simulink model "pixhawk_position_v100"  (R2016b)
settings: Solver=FixedStepAuto  StartTime=0.0  StopTime=inf  FixedStep=0.01  RelTol=1e-3
PreLoadFcn:
  | load('bus_mavlink_att_pos_mocap_t.mat');
  | load('bus_mavlink_attitude_t.mat');
  | load('bus_mavlink_heartbeat_t.mat');
  | load('bus_mavlink_raw_imu_t.mat');
  | load('bus_mavlink_set_attitude_target_t.mat');
  | load('bus_mavlink_set_mode_t.mat');
  | load('bus_mavlink_set_position_target_local_ned_t.mat');
  | 
  | load('bus_mavlink_data_stream_t.mat');
  | load('bus_mavlink_request_data_stream_t.mat');
  | load('bus_mavlink_attitude_target_t.mat');
  | load('bus_mavlink_position_target_local_ned_t.mat');
  | load('bus_mavlink_rc_channels_raw_t.mat');
  | load('bus_mavlink_rc_channels_t.mat')
libraries: dspnetwork x5, etargetslib x4, aerolibanimutils x1
settings Model: Creator=Admin  LastModifiedBy=luminghua

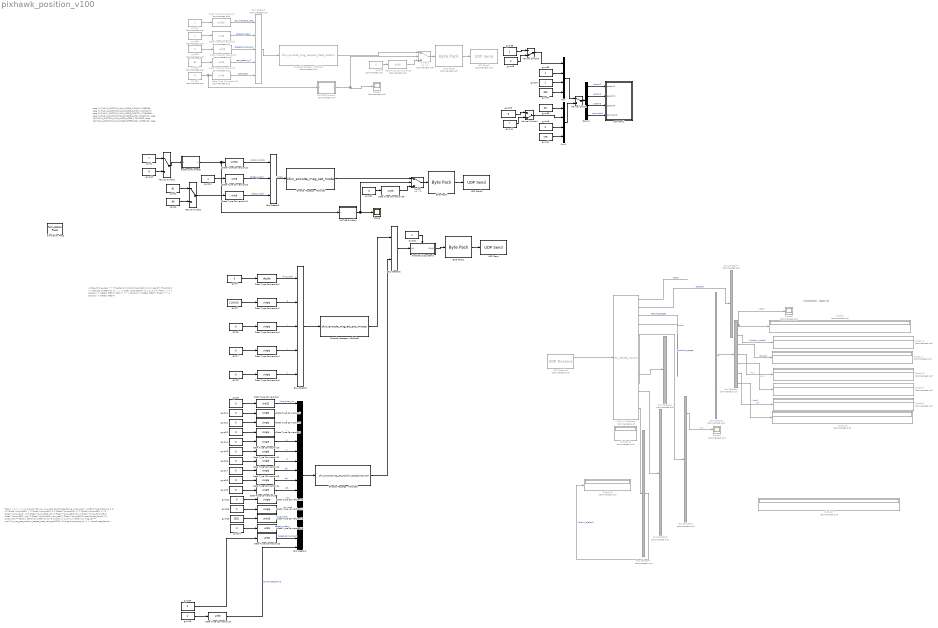
== system pixhawk_position_v100 ==
  note: case {1}%PX4_CUSTOM_MAIN_MODE_MANUAL
      |         y=65536;
      |      case {2}%PX4_CUSTOM_MAIN_MODE_ALTCTL
      |         y=131072;
      |      case {3}%PX4_CUSTOM_MAIN_MODE_POSCTL
      |         y=196608;
      |      case {4}%PX4_CUSTOM_MAIN_MODE_AUTO
      |         y=262144;
      |      case {5}%PX4_CUSTOM_MAIN_MODE_ACRO
      |         y=327680;
      |      case {6}%PX4_CUSTOM_MAIN_MODE_OFFBOARD
      |         y=393216;
      |      case {7}%PX4_CUSTOM_MAIN_MODE_STABILIZED
      |         y=458752;
      |       case {8}%PX4_CUSTOM_MAIN_MODE_RATTITUDE
  note: 不能接受数据时，查看防火墙
  note: uint64_t time_usec; /*< Timestamp (micros since boot or Unix epoch)*/
      |  float q[4]; /*< Attitude quaternion (w, x, y, z order, zero-rotation is 1, 0, 0, 0)*/
      |  float x; /*< X position in meters (NED)*/
      |  float y; /*< Y position in meters (NED)*/
      |  float z; /*< Z position in meters (NED)*/
  note: float x,y,z, vx ,vy,vz ,afx,afy,afz,yaw,yaw_rate,coordinate_frame, type_mask;
      | uint32_t time_boot_ms = 0;
      | x= (float) (*pInput[0]);
      | y = (float) (*pInput[1]);
      | z = (float) (*pInput[2]);
      | vx = (float) (*pInput[3]);
      | vy = (float) (*pInput[4]);
      | vz = (float) (*pInput[5]);
      | afx = (float) (*pInput[6]);
      | afy = (float) (*pInput[7]);
      | afz = (float) (*pInput[8]);
      | yaw = (float) (*pInput[9]);
      | yaw_rate = (float) (*pInput[10]);
      | coordinate_frame = 1;
      | type_mask = 2552;// 0001(yaw_rate) 0(yaw) 0 111(axyz) 111(vxyz) 000(xyz)
      | msg_len = mavlink_msg_set_position_target_local_ned_pack(255, 0,&msg,time_boot_ms, 1, 1, coordinate_frame, type_mask, x, y, z, vx, vy, vz, afx, afy, afz, yaw, yaw_rate);
      | ptrBuf = (uint8_T*) ssGetDWork(S,index);
      | ptrLen[index] = (real_T) mavlink_msg_to_send_buffer(ptrBuf, &msg);
      | type_mask = 1528;// 000 0(yaw_rate) 1(yaw) 0 111(axyz) 111(vxyz) 000(xyz)
      | setpoint: type_mask = 1528;// 0(idle) 0(loiter) 0(land) 0(takeoff) 0(yaw_rate) 1(yaw) 0 111(axyz) 111(vxyz) 000(xyz)
      | idle: type_mask = 34296;// 1(idle) 0(loiter) 0(land) 0(takeoff) 0(yaw_rate) 1(yaw) 0 111(axyz) 111(vxyz) 000(xyz)
      | takeoff: type_mask = 5624;// 0(idle) 0(loiter) 0(land) 1(takeoff) 0(yaw_rate) 1(yaw) 0 111(axyz) 111(vxyz) 000(xyz)
      | land: type_mask = 4856;// 0(idle) 0(loiter) 1(land) 0(takeoff) 0(yaw_rate) 1(yaw) 0 111(axyz) 111(vxyz) 000(xyz)
      |
      | yes_yaw no_yawrate
      | setpoint: type_mask = 2552;// 0(idle) 0(loiter) 0(land) 0(takeoff) 1(yaw_rate) 0(yaw) 0 111(axyz) 111(vxyz) 000(xyz)
  Bus Creator1 : BusCreator  Inputs=5  OutDataTypeStr=Bus: mavlink_att_pos_mocap_t
  Bus Creator2 : BusCreator  Inputs=2
  Bus Creator3 : BusCreator  Inputs=3  OutDataTypeStr=Bus: mavlink_set_mode_t
  Bus Creator4 : BusCreator  Inputs=16  OutDataTypeStr=Bus: mavlink_set_position_target_local_ned_t
  Bus Creator5 : BusCreator  Commented=on  Inputs=5  OutDataTypeStr=Bus: mavlink_request_data_stream_t
  Bus Creator6 : BusCreator  Commented=on  Inputs=4
  Bus Selector : BusSelector  Commented=on  OutputSignals=attitude.roll,heart.custom_mode,attitude_target.thrust,position_target.x,position_target.y,position_target.z,position_target.yaw
  Bus Selector1 : BusSelector  Commented=on  OutputSignals=time_boot_ms,q,body_roll_rate,body_pitch_rate,body_yaw_rate,thrust,type_mask
  Bus Selector2 : BusSelector  Commented=on  OutputSignals=time_boot_ms,x,y,z,vx,vy,vz,afx,afy,afz,yaw,yaw_rate,type_mask,coordinate_frame
  Bus Selector3 : BusSelector  Commented=on  OutputSignals=chan1_raw,chan2_raw,chan3_raw,chan4_raw,chan5_raw,chan6_raw,chan7_raw,chan8_raw
  Bus Selector4 : BusSelector  Commented=on  OutputSignals=chan1_scaled
  Bus Selector5 : BusSelector  Commented=on  OutputSignals=time_boot_ms,roll,pitch,yaw,rollspeed,pitchspeed,yawspeed
  Byte Pack1 : etargetslib/Byte Pack  datatypes={'uint8'}  byteAlign=1
  Byte Pack2 : etargetslib/Byte Pack  datatypes={'uint8'}  byteAlign=1
  Byte Pack3 : etargetslib/Byte Pack  Commented=on  datatypes={'uint8'}  byteAlign=1
  Data Type Conversion1 : DataTypeConversion  OutDataTypeStr=double
  Data Type Conversion{2..5,7..17} (15 alike) : DataTypeConversion  OutDataTypeStr=single
  Data Type Conversion18 : DataTypeConversion  OutDataTypeStr=uint16
  Data Type Conversion{19..21,23..24,28} (6 alike) : DataTypeConversion  OutDataTypeStr=uint8
  Data Type Conversion22 : DataTypeConversion  OutDataTypeStr=uint32
  Data Type Conversion{25..26,29..31} (5 alike) : DataTypeConversion  Commented=on  OutDataTypeStr=uint8
  Data Type Conversion27 : DataTypeConversion  Commented=on  OutDataTypeStr=uint16
  Data Type Conversion6 : DataTypeConversion  OutDataTypeStr=uint32
  Demux : Demux
  Display{,1..8,10} (10 alike) : Display  Commented=on
      Display8 settings: Format=long_e
  Enabled Subsystem1 : Subsystem  TreatAsAtomicUnit=on
  Encode Message - Attitude1 : S-Function  FunctionName=sfun_encode_msg_set_mode  SFunctionDeploymentMode=off  EnableBusSupport=off
  Encode Message - Attitude2 : S-Function  FunctionName=sfun_encode_msg_att_pos_mocap  SFunctionDeploymentMode=off  EnableBusSupport=off
  Encode Message - Attitude3 : S-Function  FunctionName=sfun_encode_msg_set_position_target_local_ned  SFunctionDeploymentMode=off  EnableBusSupport=off
  Encode Message - Attitude4 : S-Function  Commented=on  FunctionName=sfun_encode_msg_request_data_stream  SFunctionDeploymentMode=off  EnableBusSupport=off
  MATLAB Function : MATLAB Function  TreatAsAtomicUnit=on
  MATLAB Function1 : MATLAB Function  Commented=on  TreatAsAtomicUnit=on
  MAVLink Decoder2 : S-Function  Commented=on  FunctionName=sfun_decode_mavlink  SFunctionDeploymentMode=off  EnableBusSupport=off
  Manual Switch : ManualSwitch
  Manual Switch1 : ManualSwitch
  Manual Switch2 : ManualSwitch
  Manual Switch3 : ManualSwitch  CurrentSetting=0
  Manual Switch4 : ManualSwitch  CurrentSetting=0
  Mux : Mux
  Mux1 : Mux
  Scope : Scope
  Scope1 : Scope  Commented=on
  Scope2 : Scope  Commented=on
  Scope3 : Scope  Commented=on
  Simulation Pace : aerolibanimutils/Simulation Pace  SimulationPace=1  SleepMode=MATLAB Thread  OutputPaceError=off  SampleTime=0.01
  Switch : Switch  Criteria=u2 > Threshold
  Switch1 : Switch  Commented=on  Criteria=u2 > Threshold
  UDP Receive2 : dspnetwork/UDP Receive  Commented=on  localURL='0.0.0.0'  localPort=14550  remoteURL='192.168.1.101'  remotePort=-1  recvBufferSize=8192  dims=263  signalDatatype=uint8  isVarSize=off  showBlockingTime=on  blockingTime=0  sampletime=0.01  blockPlatform=HOST
  UDP Send : dspnetwork/UDP Send  remoteURL='192.168.1.100'  remotePort=14551  localURL='0.0.0.0'  localPortSource=Automatically determine  localPort=-1  sampletime=-1  blockPlatform=HOST  separateLengthPort=0
  UDP Send1 : dspnetwork/UDP Send  remoteURL='192.168.1.100'  remotePort=14551  localURL='0.0.0.0'  localPortSource=Automatically determine  localPort=-1  sampletime=-1  blockPlatform=HOST  separateLengthPort=0
  UDP Send2 : dspnetwork/UDP Send  Commented=on  remoteURL='192.168.1.101'  remotePort=14551  localURL='0.0.0.0'  localPortSource=Specify via dialog  localPort=14550  sampletime=-1  blockPlatform=HOST  separateLengthPort=0
  "command " : Subsystem
  custom_mainmode : MATLAB Function  TreatAsAtomicUnit=on
  gyro1 : Constant  Value=7  SampleTime=-1
  gyro{10,35..37} (4 alike) : Constant  SampleTime=-1
  gyro{4,6..9,11..19,21..22,24..25,31} (19 alike) : Constant  Value=0  SampleTime=0.01
  gyro2 : Constant  Value=81  SampleTime=0.01
  gyro20 : Constant  Value=6  SampleTime=-1
  gyro23 : Constant  Value=2552  SampleTime=0.01
  gyro26 : Constant  SampleTime=0.01
  gyro27 : Constant  Commented=on  SampleTime=0.01
  gyro28 : Constant  Commented=on  Value=30  SampleTime=0.01
  gyro29 : Constant  Commented=on  Value=0  SampleTime=0.01
  gyro3 : Constant  Value=80  SampleTime=0.01
  gyro30 : Constant  Commented=on  SampleTime=0.01
  gyro32 : Constant  SampleTime=0.01
  gyro33 : Constant  Commented=on  Value=0  SampleTime=0.01
  gyro34 : Constant  Commented=on  Value=0  SampleTime=0.01
  gyro38 : Constant  Value=81  SampleTime=-1
  gyro39 : Constant  Value=6  SampleTime=-1
  gyro40 : Constant  Value=0  SampleTime=-1
  gyro41 : Constant  Value=176  SampleTime=-1
  gyro42 : Constant  Value=400  SampleTime=-1
  gyro43 : Constant  Value=0  SampleTime=-1
  gyro44 : Constant  Value=7  SampleTime=-1
  gyro5 : Constant  Value=[1;0;0;0]  SampleTime=0.01
  wires:
  ? -> ?
  Encode Message - Attitude1/1 -> Switch/1
  Bus Creator3/1 -> Encode Message - Attitude1/1  "mode"
  gyro10/1 -> Data Type Conversion20/1
  Manual Switch1/1 -> Data Type Conversion21/1
  Data Type Conversion21/1 -> Bus Creator3/3  "base_mode"
  Data Type Conversion20/1 -> Bus Creator3/2  "target_system"
  Data Type Conversion22/1 -> Bus Creator3/1  "custom_mode"
  Byte Pack1/1 -> UDP Send/1
  custom_mainmode/1(y) -> MATLAB Function/1(u), Data Type Conversion22/1
  gyro2/1 -> Manual Switch1/1
  gyro3/1 -> Manual Switch1/2
  UDP Receive2/1 -> MAVLink Decoder2/1
  ? -> Display10/1
  MAVLink Decoder2/1 -> ?  "heart"
  Bus Creator1/1 -> Encode Message - Attitude2/1
  Data Type Conversion1/1 -> Bus Creator1/1  "time_usec"
  Data Type Conversion2/1 -> Bus Creator1/2  "q"
  Data Type Conversion3/1 -> Bus Creator1/3  "x"
  Data Type Conversion4/1 -> Bus Creator1/4  "y"
  Data Type Conversion5/1 -> Bus Creator1/5  "z"
  gyro4/1 -> Data Type Conversion1/1
  gyro5/1 -> Data Type Conversion2/1
  gyro6/1 -> Data Type Conversion3/1
  gyro7/1 -> Data Type Conversion4/1
  gyro8/1 -> Data Type Conversion5/1
  Encode Message - Attitude2/1 -> Bus Creator2/1
  Bus Creator2/1 -> Enabled Subsystem1/1(In1)
  Bus Creator4/1 -> Encode Message - Attitude3/1
  Data Type Conversion6/1 -> Bus Creator4/1  "time_boot_ms"
  Data Type Conversion7/1 -> Bus Creator4/2  "x"
  Data Type Conversion8/1 -> Bus Creator4/3  "y"
  Data Type Conversion9/1 -> Bus Creator4/4  "z"
  Data Type Conversion10/1 -> Bus Creator4/5  "vx"
  Data Type Conversion11/1 -> Bus Creator4/6  "vy"
  Data Type Conversion12/1 -> Bus Creator4/7  "vz"
  Data Type Conversion13/1 -> Bus Creator4/8  "afx"
  Data Type Conversion14/1 -> Bus Creator4/9  "afy"
  Data Type Conversion15/1 -> Bus Creator4/10  "afz"
  Data Type Conversion16/1 -> Bus Creator4/11  "yaw"
  Data Type Conversion17/1 -> Bus Creator4/12  "yaw_rate"
  Data Type Conversion18/1 -> Bus Creator4/13  "type_mask"
  Data Type Conversion19/1 -> Bus Creator4/14  "target_system"
  Data Type Conversion23/1 -> Bus Creator4/15  "target_component"
  Data Type Conversion24/1 -> Bus Creator4/16  "coordinate_frame"
  gyro9/1 -> Data Type Conversion6/1
  gyro11/1 -> Data Type Conversion7/1
  gyro12/1 -> Data Type Conversion8/1
  gyro13/1 -> Data Type Conversion9/1
  gyro14/1 -> Data Type Conversion10/1
  gyro15/1 -> Data Type Conversion11/1
  gyro16/1 -> Data Type Conversion12/1
  gyro17/1 -> Data Type Conversion13/1
  gyro18/1 -> Data Type Conversion14/1
  gyro19/1 -> Data Type Conversion15/1
  gyro21/1 -> Data Type Conversion16/1
  gyro22/1 -> Data Type Conversion17/1
  gyro23/1 -> Data Type Conversion18/1
  gyro24/1 -> Data Type Conversion19/1
  gyro25/1 -> Data Type Conversion23/1
  gyro26/1 -> Data Type Conversion24/1
  Encode Message - Attitude3/1 -> Bus Creator2/2
  Bus Creator5/1 -> Encode Message - Attitude4/1
  Data Type Conversion25/1 -> Bus Creator5/4  "req_stream_id"
  Data Type Conversion26/1 -> Bus Creator5/3  "target_component"
  Data Type Conversion27/1 -> Bus Creator5/1  "req_message_rate"
  gyro27/1 -> Data Type Conversion27/1
  gyro28/1 -> Data Type Conversion25/1
  MAVLink Decoder2/2 -> Bus Selector5/1  "attitude"
  Byte Pack2/1 -> UDP Send1/1
  Switch/1 -> Byte Pack2/1
  MATLAB Function/1(y) -> Scope/1, Switch/2
  Data Type Conversion28/1 -> Switch/3
  gyro31/1 -> Data Type Conversion28/1
  Enabled Subsystem1/1(Out1) -> Byte Pack1/1
  gyro32/1 -> Enabled Subsystem1/Enable
  gyro29/1 -> Data Type Conversion26/1
  gyro30/1 -> Data Type Conversion30/1
  Data Type Conversion31/1 -> Bus Creator5/5  "start_stop"
  gyro34/1 -> MATLAB Function1/1(u), Data Type Conversion31/1
  Data Type Conversion30/1 -> Bus Creator5/2  "target_system"
  Encode Message - Attitude4/1 -> Switch1/1
  Byte Pack3/1 -> UDP Send2/1
  Switch1/1 -> Byte Pack3/1
  MATLAB Function1/1(y) -> Scope1/1, Switch1/2
  Data Type Conversion29/1 -> Switch1/3
  gyro33/1 -> Data Type Conversion29/1
  Bus Creator6/1 -> Bus Selector/1
  Bus Selector/1 -> Display/1, Scope2/1  "<roll>"
  Bus Selector/2 -> Display2/1  "<custom_mode>"
  Manual Switch2/1 -> custom_mainmode/1(u)
  gyro1/1 -> Manual Switch2/1
  gyro20/1 -> Manual Switch2/2
  MAVLink Decoder2/3 -> ?  "attitude_target"
  MAVLink Decoder2/4 -> ?  "position_target"
  Bus Selector/3 -> Display1/1  "<thrust>"
  Bus Selector/4 -> Display3/1  "<x>"
  Bus Selector/5 -> Display4/1  "<y>"
  Bus Selector/6 -> Display5/1  "<z>"
  Bus Selector/7 -> Display6/1  "<yaw>"
  MAVLink Decoder2/10 -> Bus Selector1/1
  MAVLink Decoder2/11 -> Bus Selector2/1
  Bus Selector2/2 -> Scope3/1  "<x>"
  MAVLink Decoder2/12 -> Bus Selector3/1
  MAVLink Decoder2/14 -> Bus Selector4/1
  Bus Selector4/1 -> Display8/1  "<chan1_scaled>"
  ? -> ?  "confirmation"
  ? -> ?
  Demux/1 -> "command "/1(param1)  "param1"
  Demux/2 -> "command "/2(param2)  "param2"
  Demux/3 -> "command "/3(param3)  "param3"
  Demux/4 -> "command "/4(command)  "command"
  Manual Switch/1 -> Demux/1
  Mux/1 -> Manual Switch/1
  Mux1/1 -> Manual Switch/2
  gyro42/1 -> Mux/4
  gyro37/1 -> Mux/3
  gyro36/1 -> Mux/2
  Manual Switch3/1 -> Mux/1
  gyro38/1 -> Mux1/1
  Manual Switch4/1 -> Mux1/2
  gyro40/1 -> Mux1/3
  gyro41/1 -> Mux1/4
  gyro35/1 -> Manual Switch3/1
  gyro43/1 -> Manual Switch3/2
  gyro39/1 -> Manual Switch4/1
  gyro44/1 -> Manual Switch4/2

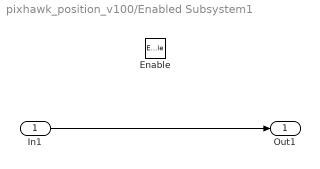
== system pixhawk_position_v100/Enabled Subsystem1 ==
  In1 : Inport
  Enable : EnablePort  StatesWhenEnabling=reset
  Out1 : Outport
  wires:
  In1/1 -> Out1/1

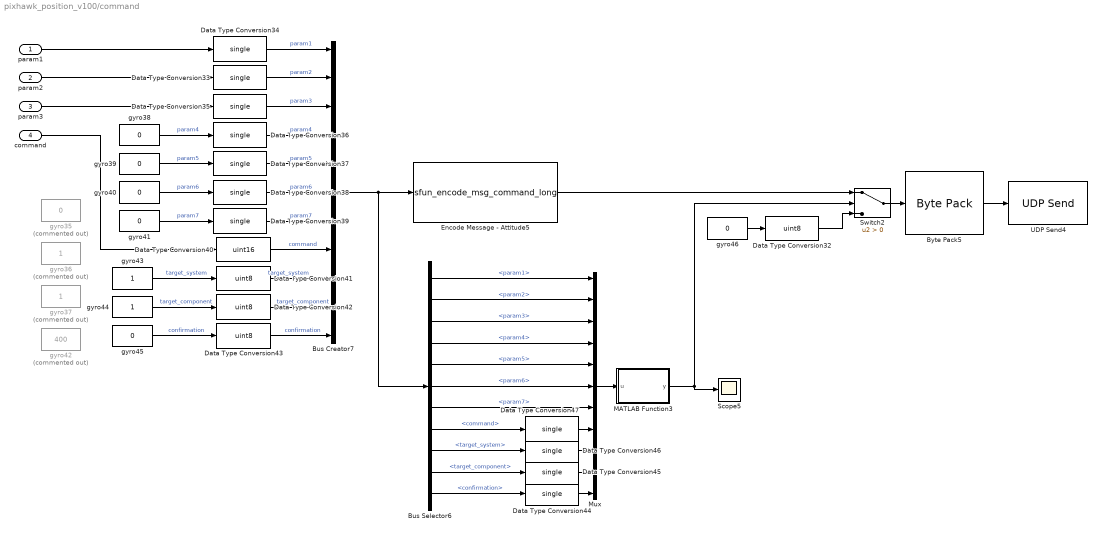
== system pixhawk_position_v100/command  ==
  param1 : Inport
  param2 : Inport  Port=2
  param3 : Inport  Port=3
  command : Inport  Port=4
  Bus Creator7 : BusCreator  Inputs=11  OutDataTypeStr=Bus: mavlink_command_long_t
  Bus Selector6 : BusSelector  OutputSignals=param1,param2,param3,param4,param5,param6,param7,command,target_system,target_component,confirmation
  Byte Pack5 : etargetslib/Byte Pack  datatypes={'uint8'}  byteAlign=1
  Data Type Conversion{32,41..43} (4 alike) : DataTypeConversion  OutDataTypeStr=uint8
  Data Type Conversion{33..39,44..47} (11 alike) : DataTypeConversion  OutDataTypeStr=single
  Data Type Conversion40 : DataTypeConversion  OutDataTypeStr=uint16
  Encode Message - Attitude5 : S-Function  FunctionName=sfun_encode_msg_command_long  SFunctionDeploymentMode=off  EnableBusSupport=off
  MATLAB Function3 : MATLAB Function  TreatAsAtomicUnit=on
  Mux : Mux  Inputs=11
  Scope5 : Scope
  Switch2 : Switch  Criteria=u2 > Threshold
  UDP Send4 : dspnetwork/UDP Send  remoteURL='192.168.1.100'  remotePort=14551  localURL='0.0.0.0'  localPortSource=Automatically determine  localPort=-1  sampletime=-1  blockPlatform=HOST  separateLengthPort=0
  gyro35 : Constant  Commented=on  Value=0  SampleTime=-1
  gyro36 : Constant  Commented=on  SampleTime=-1
  gyro37 : Constant  Commented=on  SampleTime=-1
  gyro{38..41,45} (5 alike) : Constant  Value=0  SampleTime=-1
  gyro42 : Constant  Commented=on  Value=400  SampleTime=-1
  gyro43 : Constant  SampleTime=-1
  gyro44 : Constant  SampleTime=-1
  gyro46 : Constant  Value=0  SampleTime=0.01
  wires:
  gyro43/1 -> Data Type Conversion41/1  "target_system"
  gyro44/1 -> Data Type Conversion42/1  "target_component"
  Mux/1 -> MATLAB Function3/1(u)
  Encode Message - Attitude5/1 -> Switch2/1
  Data Type Conversion43/1 -> Bus Creator7/11  "confirmation"
  Data Type Conversion42/1 -> Bus Creator7/10  "target_component"
  Data Type Conversion36/1 -> Bus Creator7/4  "param4"
  Data Type Conversion37/1 -> Bus Creator7/5  "param5"
  Data Type Conversion39/1 -> Bus Creator7/7  "param7"
  Data Type Conversion40/1 -> Bus Creator7/8  "command"
  Data Type Conversion35/1 -> Bus Creator7/3  "param3"
  Data Type Conversion33/1 -> Bus Creator7/2  "param2"
  Data Type Conversion38/1 -> Bus Creator7/6  "param6"
  Bus Creator7/1 -> Bus Selector6/1, Encode Message - Attitude5/1
  MATLAB Function3/1(y) -> Scope5/1, Switch2/2
  gyro46/1 -> Data Type Conversion32/1
  Byte Pack5/1 -> UDP Send4/1
  Switch2/1 -> Byte Pack5/1
  Data Type Conversion32/1 -> Switch2/3
  gyro41/1 -> Data Type Conversion39/1  "param7"
  gyro38/1 -> Data Type Conversion36/1  "param4"
  command/1 -> Data Type Conversion40/1
  gyro40/1 -> Data Type Conversion38/1  "param6"
  param3/1 -> Data Type Conversion35/1
  gyro39/1 -> Data Type Conversion37/1  "param5"
  gyro45/1 -> Data Type Conversion43/1  "confirmation"
  Data Type Conversion47/1 -> Mux/8
  Data Type Conversion44/1 -> Mux/11
  param1/1 -> Data Type Conversion34/1
  Data Type Conversion34/1 -> Bus Creator7/1  "param1"
  param2/1 -> Data Type Conversion33/1
  Data Type Conversion41/1 -> Bus Creator7/9  "target_system"
  Data Type Conversion46/1 -> Mux/9
  Bus Selector6/6 -> Mux/6  "<param6>"
  Bus Selector6/8 -> Data Type Conversion47/1  "<command>"
  Bus Selector6/2 -> Mux/2  "<param2>"
  Bus Selector6/1 -> Mux/1  "<param1>"
  Bus Selector6/9 -> Data Type Conversion46/1  "<target_system>"
  Bus Selector6/11 -> Data Type Conversion44/1  "<confirmation>"
  Bus Selector6/4 -> Mux/4  "<param4>"
  Bus Selector6/5 -> Mux/5  "<param5>"
  Bus Selector6/3 -> Mux/3  "<param3>"
  Bus Selector6/7 -> Mux/7  "<param7>"
  Bus Selector6/10 -> Data Type Conversion45/1  "<target_component>"
  Data Type Conversion45/1 -> Mux/10

== matlab function pixhawk_position_v100/MATLAB Function1 ==
  data: u input; y output
function y = fcn(u)
persistent u_old;
if (isempty(u_old))
    u_old = u;
end

persistent y_out;
if (isempty(y_out))
    y_out = 0;
end

if (u~=u_old)
    y_out = 1;
else
    y_out = 0;
end
u_old = u;
y = y_out;

== matlab function pixhawk_position_v100/MATLAB Function ==
  data: u input; y output
function y = fcn(u)
persistent u_old;
if (isempty(u_old))
    u_old = u;
end

persistent y_out;
if (isempty(y_out))
    y_out = 0;
end

if (u~=u_old)
    y_out = 1;
else
    y_out = 0;
end
u_old = u;
y = y_out;

== matlab function pixhawk_position_v100/custom_mainmode ==
  data: u input; y output
function y = fcn(u)
% * @file px4_custom_mode.h
 y=458752;
switch u
    case {1}%PX4_CUSTOM_MAIN_MODE_MANUAL
        y=65536;
     case {2}%PX4_CUSTOM_MAIN_MODE_ALTCTL
        y=131072;
     case {3}%PX4_CUSTOM_MAIN_MODE_POSCTL
        y=196608;
     case {4}%PX4_CUSTOM_MAIN_MODE_AUTO
        y=262144;
     case {5}%PX4_CUSTOM_MAIN_MODE_ACRO
        y=327680;
     case {6}%PX4_CUSTOM_MAIN_MODE_OFFBOARD
        y=393216;
     case {7}%PX4_CUSTOM_MAIN_MODE_STABILIZED
        y=458752;
      case {8}%PX4_CUSTOM_MAIN_MODE_RATTITUDE
        y=524288;
      
end

== matlab function pixhawk_position_v100/command /MATLAB Function3 ==
  data: u input; y output
function y = fcn(u)
persistent u_old;
if (isempty(u_old))
    u_old = u;
end

persistent y_out;
if (isempty(y_out))
    y_out = 0;
end
a_temp = (u - u_old);
if (norm(a_temp) ~= 0)
    y_out = 1;
else
    y_out = 0;
end
u_old = u;
y = y_out;
